simulink model "TPS_SWC"  (R2022b)
settings: Solver=VariableStepAuto  StartTime=0.0  StopTime=10  RelTol=1e-3
settings Model: Creator=yasso  LastModifiedBy=yasso

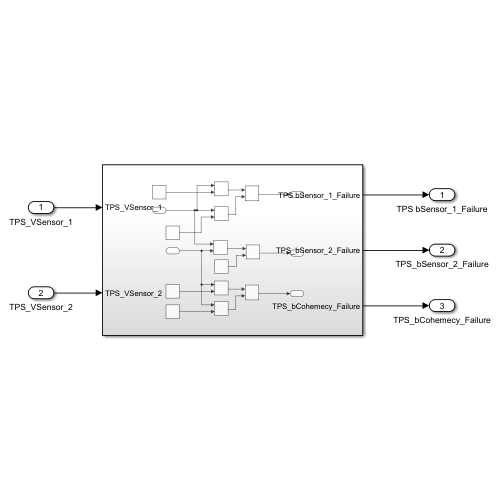
[thumbnail: Simulink's stored preview of the top-level diagram]
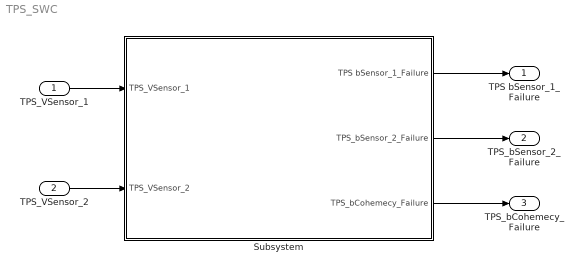
== system TPS_SWC ==
  TPS_VSensor_1 : Inport  OutDataTypeStr=single
  TPS_VSensor_2 : Inport  Port=2  OutDataTypeStr=single
  Subsystem : Subsystem
  TPS bSensor_1_Failure : Outport  OutDataTypeStr=boolean
  TPS_bSensor_2_Failure : Outport  Port=2  OutDataTypeStr=boolean
  TPS_bCohemecy_Failure : Outport  Port=3  OutDataTypeStr=boolean
  wires:
  TPS_VSensor_2/1 -> Subsystem/2(TPS_VSensor_2)
  TPS_VSensor_1/1 -> Subsystem/1(TPS_VSensor_1)
  Subsystem/1(TPS bSensor_1_Failure) -> TPS bSensor_1_Failure/1
  Subsystem/3(TPS_bCohemecy_Failure) -> TPS_bCohemecy_Failure/1
  Subsystem/2(TPS_bSensor_2_Failure) -> TPS_bSensor_2_Failure/1

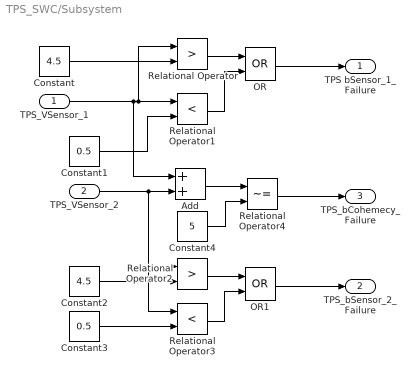
== system TPS_SWC/Subsystem ==
  TPS_VSensor_1 : Inport  OutDataTypeStr=single
  TPS_VSensor_2 : Inport  Port=2  OutDataTypeStr=single
  Add : Sum
  Constant : Constant  Value=4.5
  Constant1 : Constant  Value=0.5
  Constant2 : Constant  Value=4.5
  Constant3 : Constant  Value=0.5
  Constant4 : Constant  Value=5
  OR : Logic  Operator=OR  AllPortsSameDT=off  OutDataTypeStr=boolean
  OR1 : Logic  Operator=OR  AllPortsSameDT=off  OutDataTypeStr=boolean
  Relational Operator : RelationalOperator  Operator=>  OutDataTypeStr=boolean  RndMeth=Simplest  InputSameDT=off
  Relational Operator1 : RelationalOperator  Operator=<  OutDataTypeStr=boolean  RndMeth=Simplest  InputSameDT=off
  Relational Operator2 : RelationalOperator  Operator=>  OutDataTypeStr=boolean  RndMeth=Simplest  InputSameDT=off
  Relational Operator3 : RelationalOperator  Operator=<  OutDataTypeStr=boolean  RndMeth=Simplest  InputSameDT=off
  Relational Operator4 : RelationalOperator  Operator=~=  OutDataTypeStr=boolean  RndMeth=Simplest  InputSameDT=off
  TPS bSensor_1_Failure : Outport  OutDataTypeStr=boolean
  TPS_bSensor_2_Failure : Outport  Port=2  OutDataTypeStr=boolean
  TPS_bCohemecy_Failure : Outport  Port=3  OutDataTypeStr=boolean
  wires:
  Relational Operator1/1 -> OR/2
  Relational Operator/1 -> OR/1
  Constant/1 -> Relational Operator/2
  Constant1/1 -> Relational Operator1/2
  TPS_VSensor_1/1 -> Relational Operator/1, Relational Operator1/1, Add/1
  TPS_VSensor_2/1 -> Relational Operator3/1, Relational Operator2/1, Add/2
  Constant3/1 -> Relational Operator3/2
  Constant2/1 -> Relational Operator2/2
  Add/1 -> Relational Operator4/1
  Constant4/1 -> Relational Operator4/2
  Relational Operator2/1 -> OR1/1
  Relational Operator3/1 -> OR1/2
  OR/1 -> TPS bSensor_1_Failure/1
  Relational Operator4/1 -> TPS_bCohemecy_Failure/1
  OR1/1 -> TPS_bSensor_2_Failure/1
